simulink model "v13_T_flipflops"  (R2019b)
settings: Solver=FixedStepAuto  StartTime=0.0  StopTime=inf  FixedStep=1  MaxStep=1  RelTol=1e-3
libraries: simulink_extras x2
settings Model: Creator=MARAT  LastModifiedBy=Marat
settings SFSimCC: CustomCodeUndefinedFunction=UseInterfaceOnly

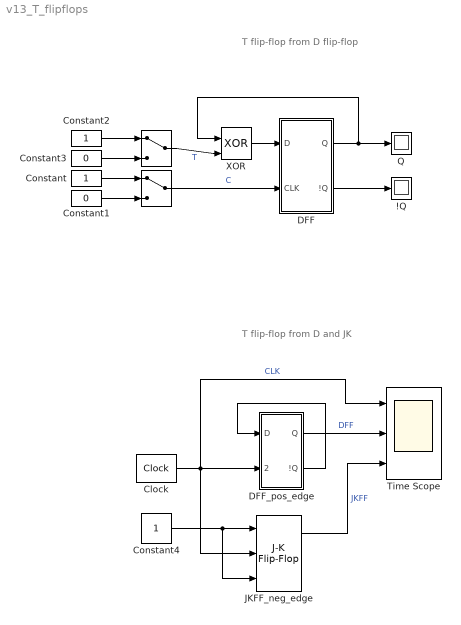
== system v13_T_flipflops ==
  note: T flip-flop from D flip-flop
  note: T flip-flop from D and JK
  " " : ManualSwitch
  " " : ManualSwitch
  !Q : Display
  Clock : simulink_extras/Flip Flops/Clock  period=2
  Constant : Constant  OutDataTypeStr=boolean
  Constant1 : Constant  Value=0  OutDataTypeStr=boolean
  Constant2 : Constant  OutDataTypeStr=boolean
  Constant3 : Constant  Value=0  OutDataTypeStr=boolean
  Constant4 : Constant  OutDataTypeStr=boolean  LockScale=on
  DFF : Subsystem
  DFF_pos_edge : Subsystem
  JKFF_neg_edge : simulink_extras/Flip Flops/J-K Flip-Flop  initial_condition=0
      settings: SourceProductName=Simulink
  Q : Display
  Time Scope : Scope  NumInputPorts=3
  XOR : Logic  Operator=XOR  IconShape=distinctive  AllPortsSameDT=off  OutDataTypeStr=boolean
  wires:
  Constant1/1 -> " "/2
  Constant/1 -> " "/1
  Constant2/1 -> " "/1
  Constant3/1 -> " "/2
  " "/1 -> XOR/2  "T"
  " "/1 -> DFF/2(CLK)  "C"
  DFF/1(Q) -> XOR/1, Q/1
  DFF/2(!Q) -> !Q/1
  XOR/1 -> DFF/1(D)
  Clock/1 -> Time Scope/1, DFF_pos_edge/2(CLK), JKFF_neg_edge/2  "CLK"
  Constant4/1 -> JKFF_neg_edge/3, JKFF_neg_edge/1
  JKFF_neg_edge/1 -> Time Scope/3  "JKFF"
  DFF_pos_edge/2(!Q) -> DFF_pos_edge/1(D)
  DFF_pos_edge/1(Q) -> Time Scope/2  "DFF"

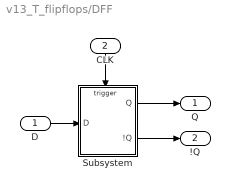
== system v13_T_flipflops/DFF ==
  D : Inport
  CLK : Inport  Port=2
  Subsystem : Subsystem
  Q : Outport  InitialOutput=0  VectorParamsAs1DForOutWhenUnconnected=off
  !Q : Outport  Port=2  InitialOutput=1  VectorParamsAs1DForOutWhenUnconnected=off
  wires:
  CLK/1 -> Subsystem/Trigger
  D/1 -> Subsystem/1(D)
  Subsystem/1(Q) -> Q/1
  Subsystem/2(!Q) -> !Q/1

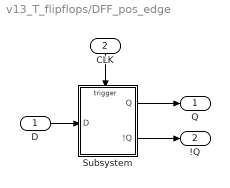
== system v13_T_flipflops/DFF_pos_edge ==
  D : Inport
  CLK : Inport  Port=2
  Subsystem : Subsystem
  Q : Outport  InitialOutput=0  VectorParamsAs1DForOutWhenUnconnected=off
  !Q : Outport  Port=2  InitialOutput=1  VectorParamsAs1DForOutWhenUnconnected=off
  wires:
  Subsystem/2(!Q) -> !Q/1
  Subsystem/1(Q) -> Q/1
  D/1 -> Subsystem/1(D)
  CLK/1 -> Subsystem/Trigger

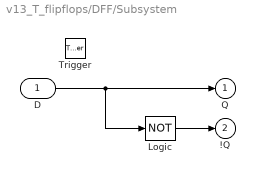
== system v13_T_flipflops/DFF/Subsystem ==
  D : Inport  LatchByDelayingOutsideSignal=on
  Trigger : TriggerPort  VariantControl=Variant  StatesWhenEnabling=reset
  Logic : Logic  Operator=NOT  Inputs=1
  Q : Outport  OutputWhenDisabled=reset  InitialOutput=0  VectorParamsAs1DForOutWhenUnconnected=off
  !Q : Outport  Port=2  OutputWhenDisabled=reset  InitialOutput=1  VectorParamsAs1DForOutWhenUnconnected=off
  wires:
  Logic/1 -> !Q/1
  D/1 -> Q/1, Logic/1

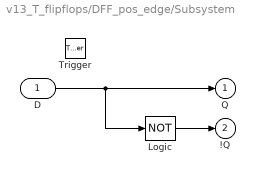
== system v13_T_flipflops/DFF_pos_edge/Subsystem ==
  D : Inport  LatchByDelayingOutsideSignal=on
  Trigger : TriggerPort  VariantControl=Variant  StatesWhenEnabling=reset
  Logic : Logic  Operator=NOT  Inputs=1
  Q : Outport  OutputWhenDisabled=reset  InitialOutput=0  VectorParamsAs1DForOutWhenUnconnected=off
  !Q : Outport  Port=2  OutputWhenDisabled=reset  InitialOutput=1  VectorParamsAs1DForOutWhenUnconnected=off
  wires:
  D/1 -> Logic/1, Q/1
  Logic/1 -> !Q/1
